simulink model "ifft_32"  (R2012b)
settings: Solver=FixedStepDiscrete  SolverMode=SingleTasking  StartTime=0.0  StopTime=2000  RelTol=1e-3
undefined symbols (not defined in the file or in its folder): Floor, Truncate
libraries: shlslibv1 x10, simulink x1
settings Model: synDspstartup=OK  Creator=sszilvasi  LastModifiedBy=sszilvasi
settings DataIOCC: SaveOutput=off  SignalLogging=off  SaveTime=off
settings OptimizationCC: InlineParams=on
settings DebuggingCC: AlgebraicLoopMsg=error

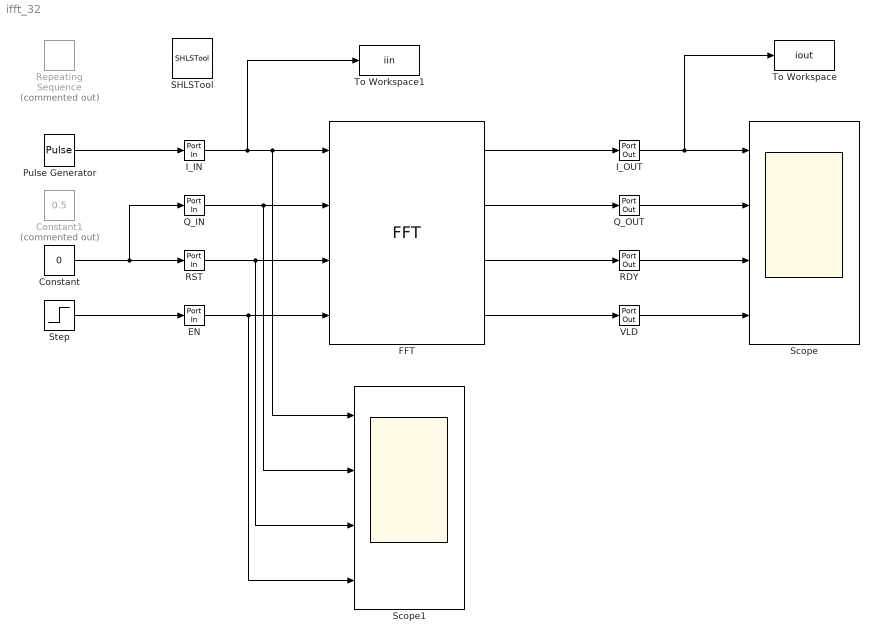
== system ifft_32 ==
  Constant : Constant  Value=0
  Constant1 : Constant  Commented=on  Value=0.5
  EN : shlslibv1/Ports & Subsystems/Port In  syn_out_wl=1  syn_out_fl=0  syn_out_dt=unsigned  syn_out_st=1  syn_capture=off  syn_register=on  syn_out_sat=off  syn_out_rnd=on  synBlockType=port  synLatency=1  synBlockId=0
  FFT : shlslibv1/Transforms/FFT  syn_fft_size=32  syn_fft_opr=Inverse  syn_real=on  syn_scale=Scale by 1/N  syn_twid_fl=10  syn_dp_f=Automatic  syn_dp_wl=syn_inp_wl  syn_dp_fl=syn_inp_fl  syn_dp_sat=off  syn_dp_round=Floor(Truncate)  syn_out_order=Natural  syn_out_f=Specify  syn_out_wl=13  syn_out_fl=12  syn_out_dt=signed  syn_out_sat=off  syn_out_round=Floor(Truncate)  syn_rst_port=on  syn_en_port=on  syn_rdy_port=on  syn_vld_port=on  synBlockType=primitive  synLatency=71  synBlockId=77
  I_IN : shlslibv1/Ports & Subsystems/Port In  syn_out_wl=4  syn_out_fl=3  syn_out_dt=signed  syn_out_st=1  syn_capture=off  syn_register=on  syn_out_sat=off  syn_out_rnd=off  synBlockType=port  synLatency=1  synBlockId=0
  I_OUT : shlslibv1/Ports & Subsystems/Port Out  syn_capture=off  syn_register=on  synBlockType=port  synLatency=1  synBlockId=1
  Pulse Generator : DiscretePulseGenerator  Amplitude=double(fi(1,1,16,15))  Period=32  PulseWidth=2  PhaseDelay=32
  Q_IN : shlslibv1/Ports & Subsystems/Port In  syn_out_wl=4  syn_out_fl=3  syn_out_dt=signed  syn_out_st=1  syn_capture=off  syn_register=on  syn_out_sat=off  syn_out_rnd=on  synBlockType=port  synLatency=1  synBlockId=0
  Q_OUT : shlslibv1/Ports & Subsystems/Port Out  syn_capture=off  syn_register=on  synBlockType=port  synLatency=1  synBlockId=1
  RDY : shlslibv1/Ports & Subsystems/Port Out  syn_capture=off  syn_register=on  synBlockType=port  synLatency=1  synBlockId=1
  RST : shlslibv1/Ports & Subsystems/Port In  syn_out_wl=1  syn_out_fl=0  syn_out_dt=unsigned  syn_out_st=1  syn_capture=off  syn_register=on  syn_out_sat=off  syn_out_rnd=on  synBlockType=port  synLatency=1  synBlockId=0
  Repeating Sequence : simulink/Sources/Repeating Sequence  Commented=on  rep_seq_t=[0 : 16]  rep_seq_y=0.75*[ones(1,15) zeros(1,2)]
  SHLSTool : shlslibv1/SHLSTool  synBlockType=tool  syn_dsp_mode=FPGA
  Scope : Scope  NumInputPorts=4
      settings: YMin=-5~-5~-5~-5  YMax=5~5~5~5
  Scope1 : Scope  NumInputPorts=4
      settings: YMin=-5~-5~-5~-5  YMax=5~5~5~5
  Step : Step  Time=32  SampleTime=1
  To Workspace : ToWorkspace  VariableName=iout  SampleTime=-1  SaveFormat=Timeseries
  To Workspace1 : ToWorkspace  VariableName=iin  SampleTime=-1  SaveFormat=Timeseries
  VLD : shlslibv1/Ports & Subsystems/Port Out  syn_capture=off  syn_register=on  synBlockType=port  synLatency=1  synBlockId=1
  wires:
  I_IN/1 -> To Workspace1/1, Scope1/1, FFT/1
  Q_IN/1 -> Scope1/2, FFT/2
  RST/1 -> Scope1/3, FFT/3
  EN/1 -> Scope1/4, FFT/4
  FFT/3 -> RDY/1
  FFT/4 -> VLD/1
  I_OUT/1 -> To Workspace/1, Scope/1
  Q_OUT/1 -> Scope/2
  RDY/1 -> Scope/3
  VLD/1 -> Scope/4
  Step/1 -> EN/1
  Constant/1 -> Q_IN/1, RST/1
  FFT/1 -> I_OUT/1
  FFT/2 -> Q_OUT/1
  Pulse Generator/1 -> I_IN/1
